simulink model "SimulinkFilter"  (R2022b)
settings: Solver=VariableStepAuto  StartTime=0.0  StopTime=10.0  RelTol=1e-3
libraries: dspsrcs4 x2, dsparch4 x1
settings Model: Creator=Cristian  LastModifiedBy=Cristian

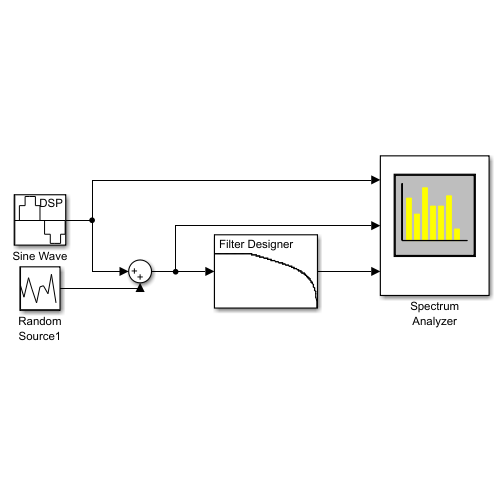
[thumbnail: Simulink's stored preview of the top-level diagram]
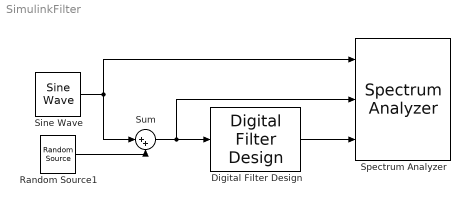
== system SimulinkFilter ==
  Digital Filter Design : dsparch4/Digital Filter Design  mwdsp_browser_bugfix_var=off
  Random Source1 : dspsrcs4/Random Source  SrcType=Uniform  NormMethod=Ziggurat  CltLength=12  MinVal=0  MaxVal=1  MeanVal=0  VarVal=1  RepMode=Not repeatable  rawSeed=1  IsInherit=off  SampMode=Discrete  SampTime=1  SampFrame=1  DataType=Double  OutComplex=Real  OutputFrames=off
  Sine Wave : dspsrcs4/Sine Wave  Amplitude=1  Frequency=100  Phase=0  SampleMode=Discrete  OutComplex=Real  CompMethod=Trigonometric fcn  TableSize=Speed  SampleTime=1/1000  SamplesPerFrame=1  ResetState=Restart at time zero  OutputFrames=off  dataType=double  wordLen=16  udDataType=sfix(16)  fracBitsMode=Best precision  numFracBits=15  OutDataTypeStr=double  LastOutDataTypeStr=double
  Spectrum Analyzer : SpectrumAnalyzer  NumInputPorts=3
  Sum : Sum  Inputs=|++
  wires:
  Sum/1 -> Digital Filter Design/1, Spectrum Analyzer/2
  Sine Wave/1 -> Sum/1, Spectrum Analyzer/1
  Random Source1/1 -> Sum/2
  Digital Filter Design/1 -> Spectrum Analyzer/3
